simulink model "JACOBIAN_01"  (R2021a)
settings: Solver=FixedStepAuto  StartTime=0.0  StopTime=1000  FixedStep=0.01  RelTol=1e-3
settings Model: Creator=TMP  LastModifiedBy=TMP
settings SolverCC: AlgebraicLoopSolver=TrustRegion
settings DebuggingCC: SFMachineParentedDataDiag=warning

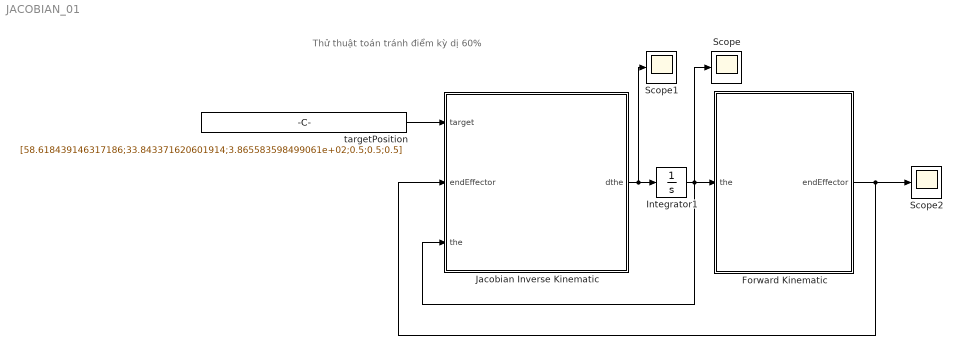
== system JACOBIAN_01 ==
  note: Thử thuật toán tránh điểm kỳ dị 60%
  Forward Kinematic : MATLAB Function  TreatAsAtomicUnit=on
  Integrator1 : Integrator  InitialCondition=[0;0;0;0;0.00001;0]
  Jacobian Inverse Kinematic : MATLAB Function  TreatAsAtomicUnit=on
  Scope : Scope
  Scope1 : Scope
  Scope2 : Scope
  targetPosition : Constant  Value=[58.618439146317186;33.843371620601914;3.865583598499061e+02;0.5;0.5;0.5]
  wires:
  targetPosition/1 -> Jacobian Inverse Kinematic/1(target)
  Integrator1/1 -> Forward Kinematic/1(the), Jacobian Inverse Kinematic/3(the), Scope/1
  Forward Kinematic/1(endEffector) -> Scope2/1, Jacobian Inverse Kinematic/2(endEffector)
  Jacobian Inverse Kinematic/1(dthe) -> Scope1/1, Integrator1/1

== matlab function JACOBIAN_01/Forward Kinematic ==
  data: the input; endEffector output
function endEffector = FK(the)
the1 = the(1);
the2 = the(2);
the3 = the(3);
the4 = the(4);
the5 = the(5);
the6 = the(6);
a1=75; a2=270; a3=90; d1=335; d4=295; d7=80;
T_0_EE = ...
[ cos(the6)*(cos(the5)*sin(the1)*sin(the4) + cos(the2 + the3)*cos(the1)*sin(the5) + cos(the1)*cos(the2)*cos(the4)*cos(the5)*sin(the3) + cos(the1)*cos(the3)*cos(the4)*cos(the5)*sin(the2)) - sin(the6)*(cos(the1)*cos(the2)*sin(the3)*sin(the4) - cos(the4)*sin(the1) + cos(the1)*cos(the3)*sin(the2)*sin(the4)), - cos(the6)*(cos(the1)*cos(the2)*sin(the3)*sin(the4) - cos(the4)*sin(the1) + cos(the1)*cos(the3)*sin(the2)*sin(the4)) - sin(the6)*(cos(the5)*sin(the1)*sin(the4) + cos(the2 + the3)*cos(the1)*sin(the5) + cos(the1)*cos(the2)*cos(the4)*cos(the5)*sin(the3) + cos(the1)*cos(the3)*cos(the4)*cos(the5)*sin(the2)), cos(the2 + the3)*cos(the1)*cos(the5) - sin(the5)*(sin(the1)*sin(the4) + cos(the1)*cos(the2)*cos(the4)*sin(the3) + cos(the1)*cos(the3)*cos(the4)*sin(the2)), a1*cos(the1) + a2*cos(the1)*sin(the2) + d4*cos(the1)*cos(the2)*cos(the3) + a3*cos(the1)*cos(the2)*sin(the3) + a3*cos(the1)*cos(the3)*sin(the2) - d4*cos(the1)*sin(the2)*sin(the3) - d7*sin(the1)*sin(the4)*sin(the5) + d7*cos(the1)*cos(the2)*cos(the3)*cos(the5) - d7*cos(the1)*cos(the5)*sin(the2)*sin(the3) - d7*cos(the1)*cos(the2)*cos(the4)*sin(the3)*sin(the5) - d7*cos(the1)*cos(the3)*cos(the4)*sin(the2)*sin(the5);
  cos(the6)*(cos(the2 + the3)*sin(the1)*sin(the5) - cos(the1)*cos(the5)*sin(the4) + cos(the2)*cos(the4)*cos(the5)*sin(the1)*sin(the3) + cos(the3)*cos(the4)*cos(the5)*sin(the1)*sin(the2)) - sin(the6)*(cos(the1)*cos(the4) + cos(the2)*sin(the1)*sin(the3)*sin(the4) + cos(the3)*sin(the1)*sin(the2)*sin(the4)), - cos(the6)*(cos(the1)*cos(the4) + cos(the2)*sin(the1)*sin(the3)*sin(the4) + cos(the3)*sin(the1)*sin(the2)*sin(the4)) - sin(the6)*(cos(the2 + the3)*sin(the1)*sin(the5) - cos(the1)*cos(the5)*sin(the4) + cos(the2)*cos(the4)*cos(the5)*sin(the1)*sin(the3) + cos(the3)*cos(the4)*cos(the5)*sin(the1)*sin(the2)), cos(the2 + the3)*cos(the5)*sin(the1) - sin(the5)*(cos(the2)*cos(the4)*sin(the1)*sin(the3) - cos(the1)*sin(the4) + cos(the3)*cos(the4)*sin(the1)*sin(the2)), a1*sin(the1) + a2*sin(the1)*sin(the2) + d4*cos(the2)*cos(the3)*sin(the1) + a3*cos(the2)*sin(the1)*sin(the3) + a3*cos(the3)*sin(the1)*sin(the2) + d7*cos(the1)*sin(the4)*sin(the5) - d4*sin(the1)*sin(the2)*sin(the3) + d7*cos(the2)*cos(the3)*cos(the5)*sin(the1) - d7*cos(the5)*sin(the1)*sin(the2)*sin(the3) - d7*cos(the2)*cos(the4)*sin(the1)*sin(the3)*sin(the5) - d7*cos(the3)*cos(the4)*sin(the1)*sin(the2)*sin(the5);
                                                                                                                                                                                          - cos(the6)*(sin(the2 + the3)*sin(the5) - cos(the2 + the3)*cos(the4)*cos(the5)) - cos(the2 + the3)*sin(the4)*sin(the6),                                                                                                                                                                                             sin(the6)*(sin(the2 + the3)*sin(the5) - cos(the2 + the3)*cos(the4)*cos(the5)) - cos(the2 + the3)*cos(the6)*sin(the4),                                                                                        - sin(the2 + the3)*cos(the5) - cos(the2 + the3)*cos(the4)*sin(the5),                                                                                                                                        d1 + a2*cos(the2) + a3*cos(the2)*cos(the3) - d4*cos(the2)*sin(the3) - d4*cos(the3)*sin(the2) - a3*sin(the2)*sin(the3) - d7*cos(the2)*cos(the5)*sin(the3) - d7*cos(the3)*cos(the5)*sin(the2) - d7*cos(the2)*cos(the3)*cos(the4)*sin(the5) + d7*cos(the4)*sin(the2)*sin(the3)*sin(the5);
                                                                                                                                                                                                                                                                                                               0,                                                                                                                                                                                                                                                                                                                0,                                                                                                                                                          0,                                                                                                                                                                                                                                                                                                                                                                                                                            1];
 
r11 = T_0_EE(1,1);
r21 = T_0_EE(2,1);
r31 = T_0_EE(3,1);
r12 = T_0_EE(1,2);
r22 = T_0_EE(2,2);
r32 = T_0_EE(3,2);
r13 = T_0_EE(1,3);
r23 = T_0_EE(2,3);
r33 = T_0_EE(3,3);
px = T_0_EE(1,4);
py = T_0_EE(2,4);
pz = T_0_EE(3,4);
pitch = atan2(-r31,sqrt(r11^2+r21^2));
yaw = atan2(r21/cos(pitch),r11/cos(pitch));
roll = atan2(r32/cos(pitch),r33/cos(pitch));
endEffector = [px;py;pz;roll;pitch;yaw];
end

== matlab function JACOBIAN_01/Jacobian Inverse Kinematic ==
  data: target input; endEffector input; dthe output; the input
function dthe = JacobianIK(target,endEffector,the)
the1 = the(1);
the2 = the(2);
the3 = the(3);
the4 = the(4);
the5 = the(5);
the6 = the(6);

a1=75; a2=270; a3=90; d1=335; d4=295; d7=80;
J = ...
[ d4*sin(the1)*sin(the2)*sin(the3) - a2*sin(the1)*sin(the2) - d4*cos(the2)*cos(the3)*sin(the1) - a3*cos(the2)*sin(the1)*sin(the3) - a3*cos(the3)*sin(the1)*sin(the2) - d7*cos(the1)*sin(the4)*sin(the5) - a1*sin(the1) - d7*cos(the2)*cos(the3)*cos(the5)*sin(the1) + d7*cos(the5)*sin(the1)*sin(the2)*sin(the3) + d7*cos(the2)*cos(the4)*sin(the1)*sin(the3)*sin(the5) + d7*cos(the3)*cos(the4)*sin(the1)*sin(the2)*sin(the5), -cos(the1)*(d4*cos(the2)*sin(the3) - a3*cos(the2)*cos(the3) - a2*cos(the2) + d4*cos(the3)*sin(the2) + a3*sin(the2)*sin(the3) + d7*cos(the2)*cos(the5)*sin(the3) + d7*cos(the3)*cos(the5)*sin(the2) + d7*cos(the2)*cos(the3)*cos(the4)*sin(the5) - d7*cos(the4)*sin(the2)*sin(the3)*sin(the5)), -cos(the1)*(d4*cos(the2)*sin(the3) - a3*cos(the2)*cos(the3) + d4*cos(the3)*sin(the2) + a3*sin(the2)*sin(the3) + d7*cos(the2)*cos(the5)*sin(the3) + d7*cos(the3)*cos(the5)*sin(the2) + d7*cos(the2)*cos(the3)*cos(the4)*sin(the5) - d7*cos(the4)*sin(the2)*sin(the3)*sin(the5)), d7*sin(the5)*(cos(the1)*cos(the2)*sin(the3)*sin(the4) - cos(the4)*sin(the1) + cos(the1)*cos(the3)*sin(the2)*sin(the4)), d7*cos(the1)*sin(the2)*sin(the3)*sin(the5) - d7*cos(the1)*cos(the2)*cos(the3)*sin(the5) - d7*cos(the5)*sin(the1)*sin(the4) - d7*cos(the1)*cos(the2)*cos(the4)*cos(the5)*sin(the3) - d7*cos(the1)*cos(the3)*cos(the4)*cos(the5)*sin(the2),                                                                                                                                                          0;
  a1*cos(the1) + a2*cos(the1)*sin(the2) + d4*cos(the1)*cos(the2)*cos(the3) + a3*cos(the1)*cos(the2)*sin(the3) + a3*cos(the1)*cos(the3)*sin(the2) - d4*cos(the1)*sin(the2)*sin(the3) - d7*sin(the1)*sin(the4)*sin(the5) + d7*cos(the1)*cos(the2)*cos(the3)*cos(the5) - d7*cos(the1)*cos(the5)*sin(the2)*sin(the3) - d7*cos(the1)*cos(the2)*cos(the4)*sin(the3)*sin(the5) - d7*cos(the1)*cos(the3)*cos(the4)*sin(the2)*sin(the5), -sin(the1)*(d4*cos(the2)*sin(the3) - a3*cos(the2)*cos(the3) - a2*cos(the2) + d4*cos(the3)*sin(the2) + a3*sin(the2)*sin(the3) + d7*cos(the2)*cos(the5)*sin(the3) + d7*cos(the3)*cos(the5)*sin(the2) + d7*cos(the2)*cos(the3)*cos(the4)*sin(the5) - d7*cos(the4)*sin(the2)*sin(the3)*sin(the5)), -sin(the1)*(d4*cos(the2)*sin(the3) - a3*cos(the2)*cos(the3) + d4*cos(the3)*sin(the2) + a3*sin(the2)*sin(the3) + d7*cos(the2)*cos(the5)*sin(the3) + d7*cos(the3)*cos(the5)*sin(the2) + d7*cos(the2)*cos(the3)*cos(the4)*sin(the5) - d7*cos(the4)*sin(the2)*sin(the3)*sin(the5)), d7*sin(the5)*(cos(the1)*cos(the4) + cos(the2)*sin(the1)*sin(the3)*sin(the4) + cos(the3)*sin(the1)*sin(the2)*sin(the4)), d7*cos(the1)*cos(the5)*sin(the4) - d7*cos(the2)*cos(the3)*sin(the1)*sin(the5) + d7*sin(the1)*sin(the2)*sin(the3)*sin(the5) - d7*cos(the2)*cos(the4)*cos(the5)*sin(the1)*sin(the3) - d7*cos(the3)*cos(the4)*cos(the5)*sin(the1)*sin(the2),                                                                                                                                                          0;
                                                                                                                                                                                                                                                                                                                                                                                                                             0,              d4*sin(the2)*sin(the3) - d4*cos(the2)*cos(the3) - a3*cos(the2)*sin(the3) - a3*cos(the3)*sin(the2) - a2*sin(the2) - d7*cos(the2)*cos(the3)*cos(the5) + d7*cos(the5)*sin(the2)*sin(the3) + d7*cos(the2)*cos(the4)*sin(the3)*sin(the5) + d7*cos(the3)*cos(the4)*sin(the2)*sin(the5),              d4*sin(the2)*sin(the3) - a3*cos(the2)*sin(the3) - a3*cos(the3)*sin(the2) - d4*cos(the2)*cos(the3) - d7*cos(the2)*cos(the3)*cos(the5) + d7*cos(the5)*sin(the2)*sin(the3) + d7*cos(the2)*cos(the4)*sin(the3)*sin(the5) + d7*cos(the3)*cos(the4)*sin(the2)*sin(the5),                                                                                d7*cos(the2 + the3)*sin(the4)*sin(the5),                                                                            d7*cos(the2)*sin(the3)*sin(the5) + d7*cos(the3)*sin(the2)*sin(the5) - d7*cos(the2)*cos(the3)*cos(the4)*cos(the5) + d7*cos(the4)*cos(the5)*sin(the2)*sin(the3),                                                                                                                                                          0;
                                                                                                                                                                                                                                                                                                                                                                                                                             0,                                                                                                                                                                                                                                                                                    -sin(the1),                                                                                                                                                                                                                                                                     -sin(the1),                                                                                             cos(the2 + the3)*cos(the1),                                                                                                                                  cos(the1)*cos(the2)*sin(the3)*sin(the4) - cos(the4)*sin(the1) + cos(the1)*cos(the3)*sin(the2)*sin(the4), cos(the2 + the3)*cos(the1)*cos(the5) - sin(the5)*(sin(the1)*sin(the4) + cos(the1)*cos(the2)*cos(the4)*sin(the3) + cos(the1)*cos(the3)*cos(the4)*sin(the2));
                                                                                                                                                                                                                                                                                                                                                                                                                             0,                                                                                                                                                                                                                                                                                     cos(the1),                                                                                                                                                                                                                                                                      cos(the1),                                                                                             cos(the2 + the3)*sin(the1),                                                                                                                                  cos(the1)*cos(the4) + cos(the2)*sin(the1)*sin(the3)*sin(the4) + cos(the3)*sin(the1)*sin(the2)*sin(the4), cos(the2 + the3)*cos(the5)*sin(the1) - sin(the5)*(cos(the2)*cos(the4)*sin(the1)*sin(the3) - cos(the1)*sin(the4) + cos(the3)*cos(the4)*sin(the1)*sin(the2));
                                                                                                                                                                                                                                                                                                                                                                                                                             1,                                                                                                                                                                                                                                                                                             0,                                                                                                                                                                                                                                                                              0,                                                                                                      -sin(the2 + the3),                                                                                                                                                                                                               cos(the2 + the3)*sin(the4),                                                                                        - sin(the2 + the3)*cos(the5) - cos(the2 + the3)*cos(the4)*sin(the5)];

%%
k1 = abs(a1 + d4*cos(the2 + the3) + a3*sin(the2 + the3) + a2*sin(the2));
k2 = abs(d4*cos(the3) + a3*sin(the3));
k3 = abs(sin(the5));
lamda0 = 0.3;
eps = 0.04;
if k1 <= eps
%     lamda1 = lamda0 * (1 - sqrt(k1/eps));
    lamda1 = lamda0*eps*exp(-(k1/eps)^2);
else
    lamda1 = 0;
end
if k2 <= eps
%     lamda2 = lamda0 * (1 - sqrt(k2/eps));
    lamda2 = lamda0*eps*exp(-(k2/eps)^2);
else
    lamda2 = 0;
end
if k3 <= eps
%     lamda3 = lamda0 * (1 - sqrt(k3/eps));
    lamda3 = lamda0*eps*exp(-(k3/eps)^2);
else
    lamda3 = 0;
end
% lamda1 = 0;
% lamda2 = 0;
% lamda3 = 0;

% k1/(k1^2 + exp(-k1)*lamda1^2)
A1 = [k1/(k1^2 + lamda1^2),                              0,                             0;
                                  0,  k2/(k2^2 + lamda2^2),                             0;
                                  0,                              0, k2/(k2^2 + lamda2^2)];
B1 = ...
[                      0,                       0, 1;
                   a3/a2,                   d4/a2, 0;
 -(a3 + a2*cos(the3))/a2, -(d4 - a2*sin(the3))/a2, 0];
J11_3 = inv(A1*B1);
R_0_3 = ...
[sin(the2 + the3)*cos(the1), cos(the2 + the3)*cos(the1), -sin(the1);
 sin(the2 + the3)*sin(the1), cos(the2 + the3)*sin(the1),  cos(the1);
           cos(the2 + the3),          -sin(the2 + the3),          0];
J11_0 = R_0_3*J11_3;

A2 = k3/(k3^2 + lamda3^2);
B2 = ...
[         1,         0,         0;
          0,         0, sin(the5);
 -cos(the5), sin(the5),         0];
J22_5 = inv(A2*B2);
R_0_5 = ...
[cos(the5)*(sin(the1)*sin(the4) + cos(the1)*cos(the2)*cos(the4)*sin(the3) + cos(the1)*cos(the3)*cos(the4)*sin(the2)) + cos(the2 + the3)*cos(the1)*sin(the5), cos(the2 + the3)*cos(the1)*cos(the5) - sin(the5)*(sin(the1)*sin(the4) + cos(the1)*cos(the2)*cos(the4)*sin(the3) + cos(the1)*cos(the3)*cos(the4)*sin(the2)), cos(the1)*cos(the2)*sin(the3)*sin(the4) - cos(the4)*sin(the1) + cos(the1)*cos(the3)*sin(the2)*sin(the4);
 cos(the5)*(cos(the2)*cos(the4)*sin(the1)*sin(the3) - cos(the1)*sin(the4) + cos(the3)*cos(the4)*sin(the1)*sin(the2)) + cos(the2 + the3)*sin(the1)*sin(the5), cos(the2 + the3)*cos(the5)*sin(the1) - sin(the5)*(cos(the2)*cos(the4)*sin(the1)*sin(the3) - cos(the1)*sin(the4) + cos(the3)*cos(the4)*sin(the1)*sin(the2)), cos(the1)*cos(the4) + cos(the2)*sin(the1)*sin(the3)*sin(the4) + cos(the3)*sin(the1)*sin(the2)*sin(the4);
                                                                                          cos(the2 + the3)*cos(the4)*cos(the5) - sin(the2 + the3)*sin(the5),                                                                                        - sin(the2 + the3)*cos(the5) - cos(the2 + the3)*cos(the4)*sin(the5),                                                                              cos(the2 + the3)*sin(the4)];
J22_0 = R_0_5*J22_5;
J12_0 = J(1:3,4:6);
J21_0 = J(4:6,1:3);
J_ = [J11_0,J12_0;
      J21_0,J22_0];
n = 0.1; % tốc độ học
dthe = inv(J_)*n*(target - endEffector);
